simulink model "third_body_perturbations"  (R2023a)
settings: Solver=FixedStepAuto  StartTime=0.0  StopTime=1000.0  FixedStep=0.001  RelTol=1e-3
settings Model: Creator=orous  LastModifiedBy=orous
settings DataIOCC: ExternalInput=X_icrf,t_JD  LoadExternalInput=on

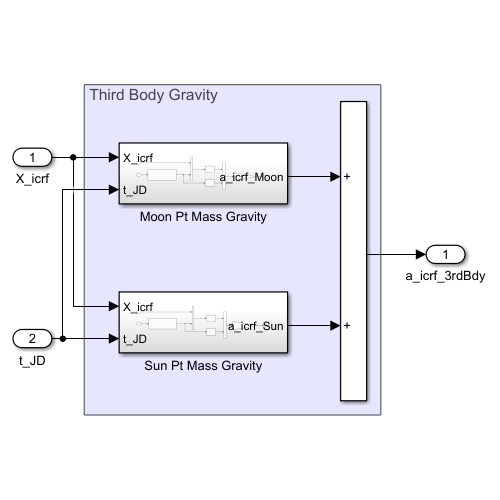
[thumbnail: Simulink's stored preview of the top-level diagram]
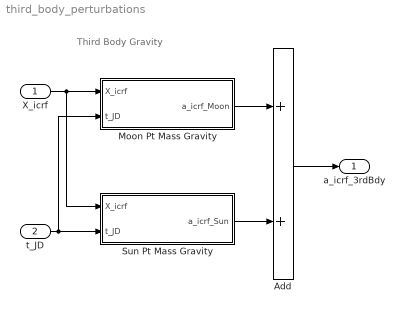
== system third_body_perturbations ==
  note: Third Body Gravity
  X_icrf : Inport  PortDimensions=3
  t_JD : Inport  Port=2  PortDimensions=1
  Add : Sum  Inputs=2
  Moon Pt Mass Gravity : Subsystem
  Sun Pt Mass Gravity : Subsystem
  a_icrf_3rdBdy : Outport
  wires:
  Moon Pt Mass Gravity/1(a_icrf_Moon) -> Add/1
  t_JD/1 -> Moon Pt Mass Gravity/2(t_JD), Sun Pt Mass Gravity/2(t_JD)
  Sun Pt Mass Gravity/1(a_icrf_Sun) -> Add/2
  X_icrf/1 -> Moon Pt Mass Gravity/1(X_icrf), Sun Pt Mass Gravity/1(X_icrf)
  Add/1 -> a_icrf_3rdBdy/1

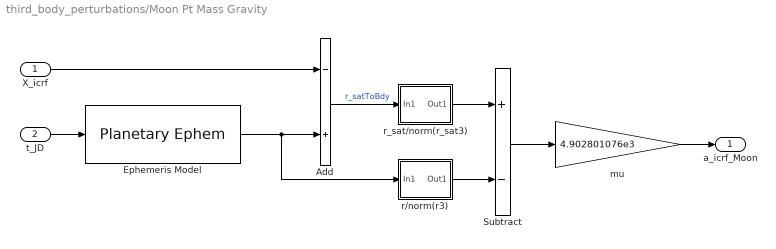
== system third_body_perturbations/Moon Pt Mass Gravity ==
  X_icrf : Inport
  t_JD : Inport  Port=2
  Add : Sum  Inputs=-+
  Ephemeris Model : PlanetaryEphem  outputVelocity=off
      settings: AttributesFormatString=|
      | %<nCenter> to %<nTarget>
      | JPL Model: %<de>
  Subtract : Sum  Inputs=+-
  mu : Gain  Gain=4.902801076e3
  r/norm(r3) : Subsystem
  r_sat/norm(r_sat3) : Subsystem
  a_icrf_Moon : Outport
  wires:
  mu/1 -> a_icrf_Moon/1
  r_sat/norm(r_sat3)/1(Out1) -> Subtract/1
  Subtract/1 -> mu/1
  Ephemeris Model/1 -> Add/2, r/norm(r3)/1(In1)
  X_icrf/1 -> Add/1
  Add/1 -> r_sat/norm(r_sat3)/1(In1)  "r_satToBdy"
  r/norm(r3)/1(Out1) -> Subtract/2
  t_JD/1 -> Ephemeris Model/1

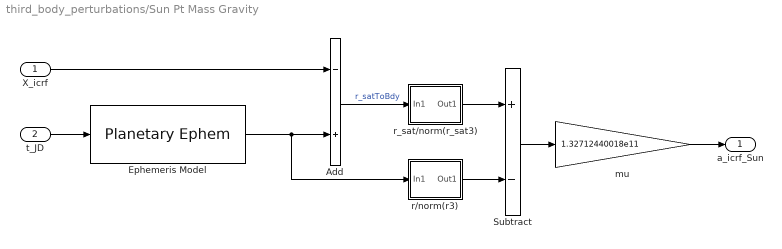
== system third_body_perturbations/Sun Pt Mass Gravity ==
  X_icrf : Inport
  t_JD : Inport  Port=2
  Add : Sum  Inputs=-+
  Ephemeris Model : PlanetaryEphem  target=Sun  outputVelocity=off
      settings: AttributesFormatString=|
      | %<nCenter> to %<nTarget>
      | JPL Model: %<de>
  Subtract : Sum  Inputs=+-
  mu : Gain  Gain=1.32712440018e11
  r/norm(r3) : Subsystem
  r_sat/norm(r_sat3) : Subsystem
  a_icrf_Sun : Outport
  wires:
  t_JD/1 -> Ephemeris Model/1
  r/norm(r3)/1(Out1) -> Subtract/2
  Add/1 -> r_sat/norm(r_sat3)/1(In1)  "r_satToBdy"
  X_icrf/1 -> Add/1
  Ephemeris Model/1 -> r/norm(r3)/1(In1), Add/2
  Subtract/1 -> mu/1
  r_sat/norm(r_sat3)/1(Out1) -> Subtract/1
  mu/1 -> a_icrf_Sun/1

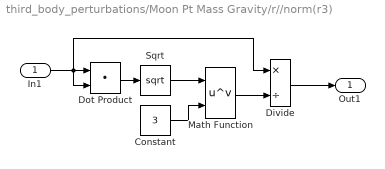
== system third_body_perturbations/Moon Pt Mass Gravity/r//norm(r3) ==
  In1 : Inport
  Constant : Constant  Value=3
  Divide : Product  Inputs=*/
  Dot Product : DotProduct  OutDataTypeStr=Inherit: Inherit via internal rule
  Math Function : Math  Operator=pow
  Sqrt : Sqrt
  Out1 : Outport
  wires:
  Math Function/1 -> Divide/2
  Constant/1 -> Math Function/2
  In1/1 -> Divide/1, Dot Product/2, Dot Product/1
  Sqrt/1 -> Math Function/1
  Dot Product/1 -> Sqrt/1
  Divide/1 -> Out1/1

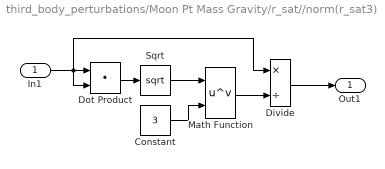
== system third_body_perturbations/Moon Pt Mass Gravity/r_sat//norm(r_sat3) ==
  In1 : Inport
  Constant : Constant  Value=3
  Divide : Product  Inputs=*/
  Dot Product : DotProduct  OutDataTypeStr=Inherit: Inherit via internal rule
  Math Function : Math  Operator=pow
  Sqrt : Sqrt
  Out1 : Outport
  wires:
  Divide/1 -> Out1/1
  Dot Product/1 -> Sqrt/1
  Sqrt/1 -> Math Function/1
  In1/1 -> Dot Product/1, Dot Product/2, Divide/1
  Constant/1 -> Math Function/2
  Math Function/1 -> Divide/2

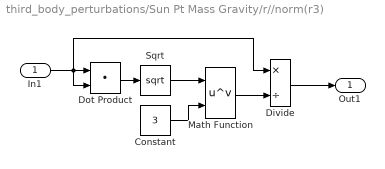
== system third_body_perturbations/Sun Pt Mass Gravity/r//norm(r3) ==
  In1 : Inport
  Constant : Constant  Value=3
  Divide : Product  Inputs=*/
  Dot Product : DotProduct  OutDataTypeStr=Inherit: Inherit via internal rule
  Math Function : Math  Operator=pow
  Sqrt : Sqrt
  Out1 : Outport
  wires:
  Divide/1 -> Out1/1
  Dot Product/1 -> Sqrt/1
  Sqrt/1 -> Math Function/1
  In1/1 -> Dot Product/1, Dot Product/2, Divide/1
  Constant/1 -> Math Function/2
  Math Function/1 -> Divide/2

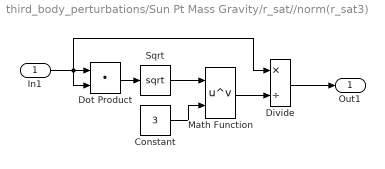
== system third_body_perturbations/Sun Pt Mass Gravity/r_sat//norm(r_sat3) ==
  In1 : Inport
  Constant : Constant  Value=3
  Divide : Product  Inputs=*/
  Dot Product : DotProduct  OutDataTypeStr=Inherit: Inherit via internal rule
  Math Function : Math  Operator=pow
  Sqrt : Sqrt
  Out1 : Outport
  wires:
  Math Function/1 -> Divide/2
  Constant/1 -> Math Function/2
  In1/1 -> Divide/1, Dot Product/2, Dot Product/1
  Sqrt/1 -> Math Function/1
  Dot Product/1 -> Sqrt/1
  Divide/1 -> Out1/1
